simulink library "csc_tlt_takeoff_landing_table_guidance_lib"  (R2015b)
settings: Solver=ode45  StartTime=0.0  StopTime=10.0  RelTol=1e-3
values from neighbouring files (symbols this model uses):
  tlt_off_vertical_limit = 5.0    (= 5)    [csc_tlt_takeoff_landing_table_guidance_init.m]
  tlt_off_vertical_limit_altitude_enable = 300    [csc_tlt_takeoff_landing_table_guidance_init.m]
  tlt_terminal_vertical_vel_zero_mean_bias = 0.00    (= 0)    [csc_tlt_takeoff_landing_table_guidance_init.m]
libraries: simulink x2, csu_tbg_table_based_guidance_lib x2, util_extra_lib x1, util_info_lib x1, util_common_lib x1
settings Model: Creator=escrane  LastModifiedBy=jimkaidy
settings DataIOCC: SaveFormat=Array
settings DebuggingCC: UnderspecifiedInitializationDetection=Classic  MergeDetectMultiDrivingBlocksExec=none  SolverPrmCheckMsg=warning
settings HardwareCC: ProdBitPerPointer=32  ProdLargestAtomicFloat=None  ProdIntDivRoundTo=Undefined  ProdEndianess=Unspecified  ProdWordSize=32  ProdHWDeviceType=32-bit Generic
settings GRTTargetCC: GeneratePreprocessorConditionals=Disable all
settings ConfigComp: CovModelRefEnable=Off  CovSFcnEnable=off

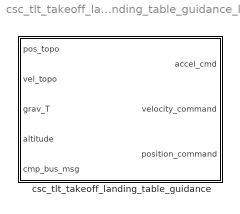
== system csc_tlt_takeoff_landing_table_guidance_lib ==
  csc_tlt_takeoff_landing_table_guidance : Subsystem  VariantControl=(default)

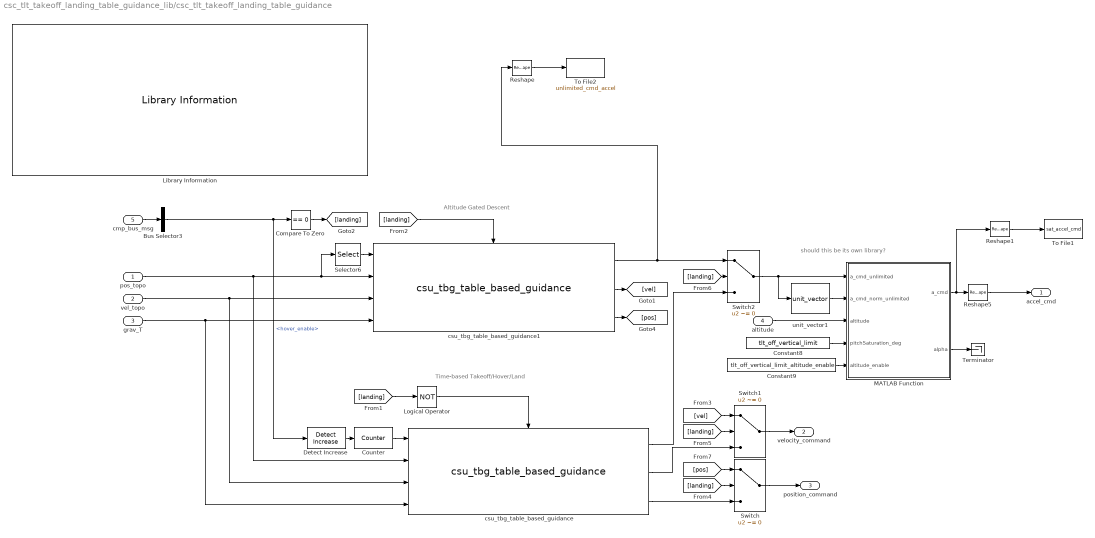
== system csc_tlt_takeoff_landing_table_guidance_lib/csc_tlt_takeoff_landing_table_guidance ==
  note: should this be its own library?
  note: Time-based Takeoff/Hover/Land
  note: Altitude Gated Descent
  pos_topo : Inport
  vel_topo : Inport  Port=2
  grav_T : Inport  Port=3
  altitude : Inport  Port=4
  cmp_bus_msg : Inport  Port=5
  Bus Selector3 : BusSelector  OutputSignals=hover_enable
  Compare To Zero : simulink/Logic and Bit Operations/Compare To Zero  relop===  OutDataTypeStr=boolean
  Constant8 : Constant  Value=tlt_off_vertical_limit  VectorParams1D=off
  Constant9 : Constant  Value=tlt_off_vertical_limit_altitude_enable  VectorParams1D=off
  Counter : util_extra_lib/Counter  dt=csc_gdn_dt  v0=0  dv=csc_gdn_dt
  Detect Increase : simulink/Logic and Bit Operations/Detect Increase  vinit=0.0  InputProcessing=Inherited  OutDataTypeStr=boolean
  Library Information : util_info_lib/Library Information  owner='NONE'
  Logical Operator : Logic  Operator=NOT  AllPortsSameDT=off  OutDataTypeStr=boolean
  MATLAB Function : MATLAB Function  TreatAsAtomicUnit=on
  Reshape : Reshape
  Reshape1 : Reshape
  Reshape5 : Reshape  OutputDimensionality=Column vector (2-D)
  Selector6 : Selector  InputPortWidth=3  IndexOptions=Index vector (dialog)  Indices=[3]  OutputSizes=1
  Switch : Switch  Criteria=u2 ~= 0
  Switch1 : Switch  Criteria=u2 ~= 0
  Switch2 : Switch  Criteria=u2 ~= 0
  Terminator : Terminator
  To File1 : ToFile  Filename=sat_accel_cmd  MatrixName=sat_accel_cmd  SaveFormat=Timeseries
  To File2 : ToFile  Filename=unlimited_cmd_accel  MatrixName=unlimited_cmd_accel  SaveFormat=Timeseries
  csu_tbg_table_based_guidance : csu_tbg_table_based_guidance_lib/csu_tbg_table_based_guidance  guidance_table=tlt_takeoff_hover_translate_table  guidance_table_num_entries=tlt_takeoff_hover_translate_table_length  entry_comparison=>=  velocity_bias=[0 0 tlt_terminal_vertical_vel_zero_mean_bias]
  csu_tbg_table_based_guidance1 : csu_tbg_table_based_guidance_lib/csu_tbg_table_based_guidance  guidance_table=tlt_descent_translate_table  guidance_table_num_entries=tlt_descent_translate_table_length  entry_comparison=<  velocity_bias=[0 0 tlt_terminal_vertical_vel_zero_mean_bias]
  unit_vector1 : util_common_lib/unit_vector  SystemSampleTime=-1
  accel_cmd : Outport
  velocity_command : Outport  Port=2
  position_command : Outport  Port=3
  wires:
  [landing] -> Switch2/2
  [landing] -> Switch1/2
  [landing] -> Switch/2
  [landing] -> csu_tbg_table_based_guidance1/Enable
  Logical Operator/1 -> csu_tbg_table_based_guidance/Enable
  [landing] -> Logical Operator/1
  Compare To Zero/1 -> [landing]
  Switch/1 -> position_command/1
  Switch1/1 -> velocity_command/1
  [vel] -> Switch1/1
  csu_tbg_table_based_guidance1/2 -> [vel]
  csu_tbg_table_based_guidance1/3 -> [pos]
  [pos] -> Switch/1
  csu_tbg_table_based_guidance/2 -> Switch1/3
  csu_tbg_table_based_guidance/3 -> Switch/3
  Bus Selector3/1 -> Detect Increase/1, Compare To Zero/1  "<hover_enable>"
  csu_tbg_table_based_guidance/1 -> Switch2/3
  csu_tbg_table_based_guidance1/1 -> Reshape/1, Switch2/1
  grav_T/1 -> csu_tbg_table_based_guidance/4, csu_tbg_table_based_guidance1/4
  vel_topo/1 -> csu_tbg_table_based_guidance/3, csu_tbg_table_based_guidance1/3
  pos_topo/1 -> csu_tbg_table_based_guidance/2, Selector6/1, csu_tbg_table_based_guidance1/2
  Selector6/1 -> csu_tbg_table_based_guidance1/1
  Detect Increase/1 -> Counter/1
  Counter/1 -> csu_tbg_table_based_guidance/1
  altitude/1 -> MATLAB Function/3(altitude)
  Constant9/1 -> MATLAB Function/5(altitude_enable)
  MATLAB Function/2(alpha) -> Terminator/1
  Reshape5/1 -> accel_cmd/1
  Switch2/1 -> unit_vector1/1, MATLAB Function/1(a_cmd_unlimited)
  MATLAB Function/1(a_cmd) -> Reshape1/1, Reshape5/1
  Constant8/1 -> MATLAB Function/4(pitchSaturation_deg)
  unit_vector1/1 -> MATLAB Function/2(a_cmd_norm_unlimited)
  cmp_bus_msg/1 -> Bus Selector3/1
  Reshape/1 -> To File2/1
  Reshape1/1 -> To File1/1

== matlab function csc_tlt_takeoff_landing_table_guidance_lib/csc_tlt_takeoff_landing_table_guidance/MATLAB Function ==
  data: a_cmd_unlimited input; a_cmd_norm_unlimited input; altitude input; a_cmd output; pitchSaturation_deg input; alpha output; altitude_enable input
function [a_cmd, alpha] = PitchSaturation(a_cmd_unlimited,a_cmd_norm_unlimited,altitude,pitchSaturation_deg,altitude_enable)
%#codegen


a_cmd = zeros(1,3);
X1 = 0.0;
Y1 = 0.0;

X2 = a_cmd_norm_unlimited(1);
Y2 = a_cmd_norm_unlimited(2);
Z2 = a_cmd_norm_unlimited(3);   

% this is no longer a magnitude
a_cmd_mag = a_cmd_unlimited(3);

alpha = acosd(Z2);

if alpha > 90
    alpha = 90;
    a_cmd_mag = 0;
end

if (alpha >= pitchSaturation_deg) && (altitude <= altitude_enable)
    
    if abs(X2) >= 1e-9 && abs(Y2) < 1e-9
        X1 = sind(pitchSaturation_deg);
        Y1 = 0.0;
    elseif abs(X2) < 1e-9 && abs(Y2) >= 1e-9
        X1 = 0.0;
        Y1 = sind(pitchSaturation_deg);    
    elseif abs(X2) < 1e-9 && abs(Y2) < 1e-9
        X1 = 0.0;
        Y1 = 0.0;    
    elseif abs(X2) >= 1e-9 && abs(Y2) >= 1e-9
        X1 = sqrt(((X2/Y2)^2)*(1-(cosd(pitchSaturation_deg))^2)/(1+(X2/Y2)^2));
        Y1 = abs(X1*Y2/X2);    
    end
    Z1 = cosd(pitchSaturation_deg);

    a_cmd(1,1) = X1*sign(X2);
    a_cmd(1,2) = Y1*sign(Y2);
    a_cmd(1,3) = abs(Z1);
       
else
    a_cmd(1,1) = X2;
    a_cmd(1,2) = Y2;
    a_cmd(1,3) = abs(Z2);
    
end

a_cmd = a_cmd_mag*a_cmd;
